simulink model "simx"  (R2018a)
settings: Solver=VariableStepAuto  StartTime=0.0  StopTime=10.0  RelTol=1e-3
values from neighbouring files (symbols this model uses):
  b0 = 0.005    [sol.m]
  b1 = 0.01    [sol.m]
  b2 = 0.01    [sol.m]
libraries: fuzblock x1
settings Model: Creator=daniel  LastModifiedBy=daniel

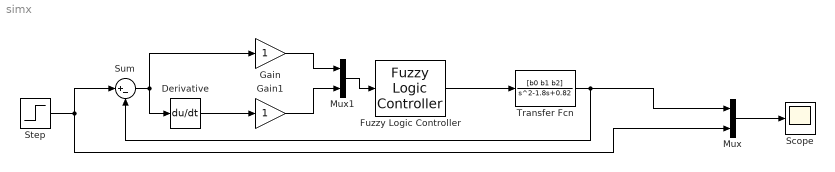
== system simx ==
  Derivative : Derivative
  Fuzzy Logic Controller : fuzblock/Fuzzy Logic  Controller  FIS=sys  OutputSampleNumber=101  DataType=double  FuzzifiedInputs=off  RuleFiringStrengths=off  RuleOutputs=off  AggregatedOutputs=off  SimulateUsing=Interpreted execution  OutOfRangeInputValueMessage=warning  NoRuleFiredMessage=warning  EmptyOutputFuzzySetMessage=warning
  Gain : Gain
  Gain1 : Gain
  Mux : Mux  Inputs=2
  Mux1 : Mux  Inputs=2
  Scope : Scope
  Step : Step  SampleTime=0
  Sum : Sum  Inputs=|+-
  Transfer Fcn : TransferFcn  Numerator=[b0 b1 b2]  Denominator=[1 -1.8 0.82]
  wires:
  Mux/1 -> Scope/1
  Step/1 -> Sum/1, Mux/2
  Transfer Fcn/1 -> Sum/2, Mux/1
  Mux1/1 -> Fuzzy Logic Controller/1
  Fuzzy Logic Controller/1 -> Transfer Fcn/1
  Sum/1 -> Gain/1, Derivative/1
  Derivative/1 -> Gain1/1
  Gain1/1 -> Mux1/2
  Gain/1 -> Mux1/1
